simulink model "LuGre"  (R2019b)
settings: Solver=ode45  StartTime=0.0  StopTime=10.0  RelTol=1e-3
settings Model: Creator=xyh  LastModifiedBy=user
settings SolverCC: ZeroCrossAlgorithm=Adaptive
settings DebuggingCC: IgnoredZcDiagnostic=none

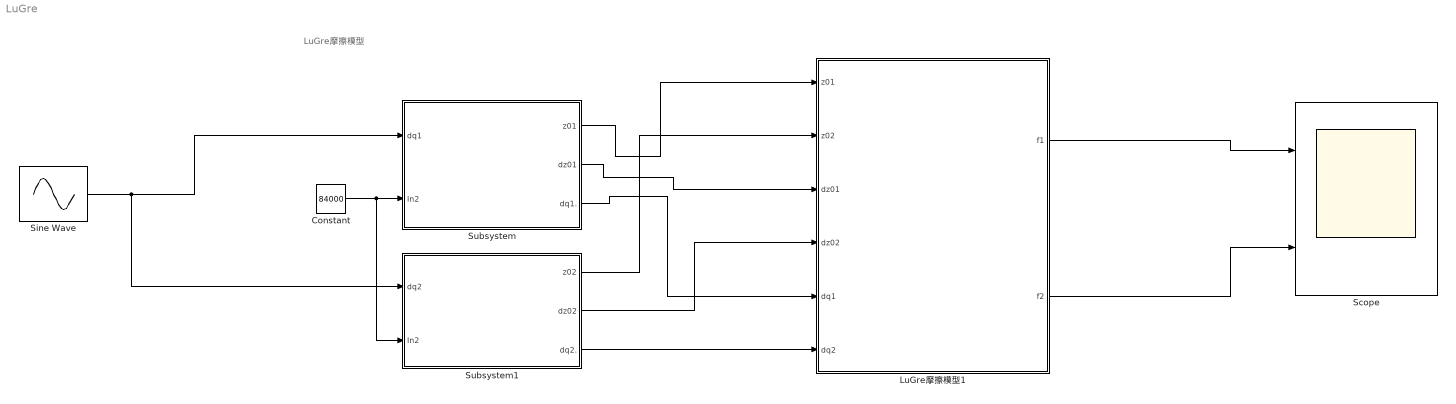
== system LuGre ==
  note: LuGre摩擦模型
  Constant : Constant  Value=84000
  LuGre摩擦模型1 : MATLAB Function  TreatAsAtomicUnit=on
  Scope : Scope  NumInputPorts=2
  Sine Wave : Sin  SampleTime=0
  Subsystem : Subsystem
  Subsystem1 : Subsystem
  wires:
  Subsystem1/3(dq2.) -> LuGre摩擦模型1/6(dq2)
  Subsystem1/2(dz02) -> LuGre摩擦模型1/4(dz02)
  Subsystem1/1(z02) -> LuGre摩擦模型1/2(z02)
  Sine Wave/1 -> Subsystem1/1(dq2), Subsystem/1(dq1)
  Subsystem/3(dq1.) -> LuGre摩擦模型1/5(dq1)
  Subsystem/2(dz01) -> LuGre摩擦模型1/3(dz01)
  Subsystem/1(z01) -> LuGre摩擦模型1/1(z01)
  Constant/1 -> Subsystem1/2(In2), Subsystem/2(In2)
  LuGre摩擦模型1/1(f1) -> Scope/1
  LuGre摩擦模型1/2(f2) -> Scope/2

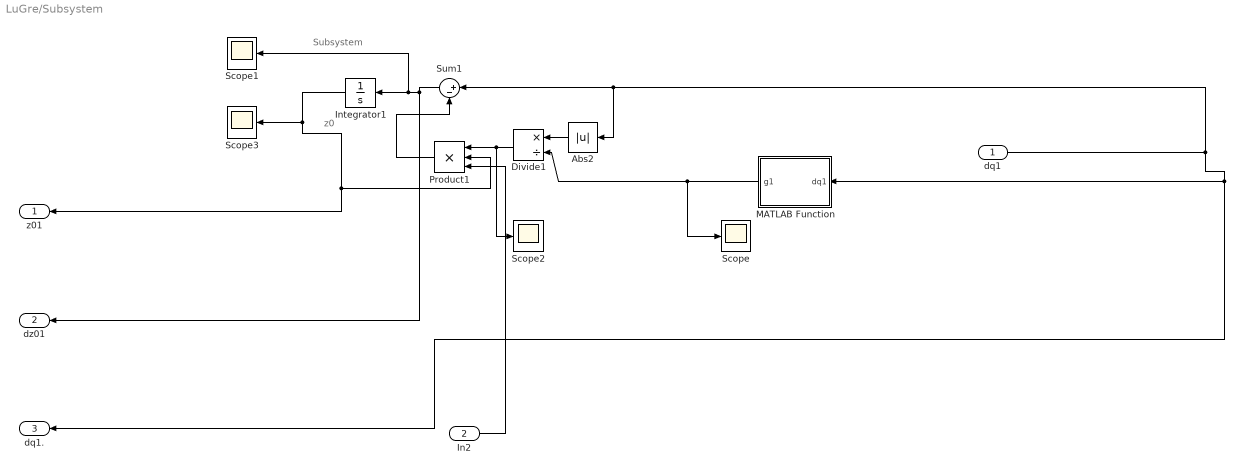
== system LuGre/Subsystem ==
  note: z0
  note: Subsystem
  dq1 : Inport
  In2 : Inport  Port=2
  Abs2 : Abs
  Divide1 : Product  Inputs=*/
  Integrator1 : Integrator
  MATLAB Function : MATLAB Function  TreatAsAtomicUnit=on
  Product1 : Product  Inputs=3
  Scope{,1..3} (4 alike) : Scope
  Sum1 : Sum  Inputs=|+-
  z01 : Outport
  dz01 : Outport  Port=2
  dq1. : Outport  Port=3
  wires:
  Product1/1 -> Sum1/2
  Abs2/1 -> Divide1/1
  Integrator1/1 -> Scope3/1, z01/1, Product1/2
  Sum1/1 -> dz01/1, Scope1/1, Integrator1/1
  Divide1/1 -> Product1/1, Scope2/1
  dq1/1 -> Abs2/1, Sum1/1, dq1./1, MATLAB Function/1(dq1)
  In2/1 -> Product1/3
  MATLAB Function/1(g1) -> Divide1/2, Scope/1

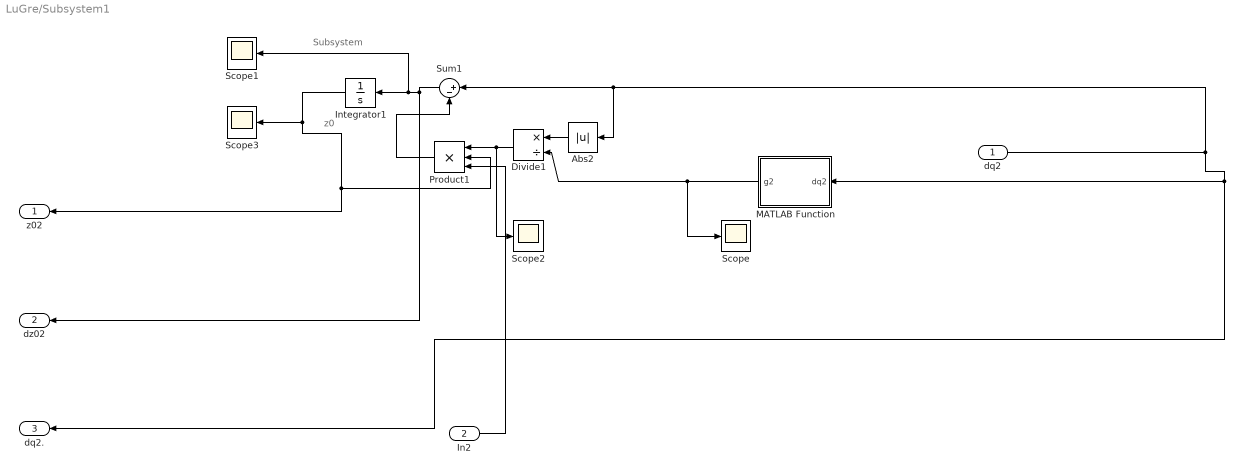
== system LuGre/Subsystem1 ==
  note: Subsystem
  note: z0
  dq2 : Inport
  In2 : Inport  Port=2
  Abs2 : Abs
  Divide1 : Product  Inputs=*/
  Integrator1 : Integrator
  MATLAB Function : MATLAB Function  TreatAsAtomicUnit=on
  Product1 : Product  Inputs=3
  Scope{,1..3} (4 alike) : Scope
  Sum1 : Sum  Inputs=|+-
  z02 : Outport
  dz02 : Outport  Port=2
  dq2. : Outport  Port=3
  wires:
  MATLAB Function/1(g2) -> Scope/1, Divide1/2
  In2/1 -> Product1/3
  dq2/1 -> MATLAB Function/1(dq2), dq2./1, Sum1/1, Abs2/1
  Divide1/1 -> Scope2/1, Product1/1
  Sum1/1 -> Integrator1/1, Scope1/1, dz02/1
  Integrator1/1 -> Product1/2, z02/1, Scope3/1
  Abs2/1 -> Divide1/1
  Product1/1 -> Sum1/2

== matlab function LuGre/Subsystem1/MATLAB Function ==
  data: dq2 input; g2 output
function g2 = fcn(dq2)
xite1 = 260;
xite2 = 28;
Fc = 3.82;
Fs = 8.16;
dqs = 0.0125;

g2 = Fc + (Fs-Fc)*exp(-(dq2/dqs)^2);

== matlab function LuGre/LuGre摩擦模型1 ==
  data: z01 input; z02 input; dz01 input; dz02 input; dq1 input; f1 output; dq2 input; f2 output
function [f1,f2] = fcn(z01,z02,dz01,dz02,dq1,dq2)
xite0 = 84000;
xite1 = 260;
xite2 = 28;
Fc = 3.82;
Fs = 8.16;
dqs = 0.0125;
lamda = 1;

f1 = lamda * (xite0 * z01 + xite1 * dz01 + xite2 * dq1);
f2 = lamda * (xite0 * z02 + xite1 * dz02 + xite2 * dq2);

== matlab function LuGre/Subsystem/MATLAB Function ==
  data: dq1 input; g1 output
function g1 = fcn(dq1)
xite1 = 260;
xite2 = 28;
Fc = 3.82;
Fs = 8.16;
dqs = 0.0125;

g1 = Fc + (Fs-Fc)*exp(-(dq1/dqs)^2);
